simulink model "VehicleDynamicsModel"  (R2018a)
settings: Solver=ode15s  StartTime=0.0  StopTime=12  FixedStep=0.01  RelTol=1e-2  EnableMultiTasking=on
PreLoadFcn:
  | PowerTrain_14DOF_ini
StopFcn:
  | AfterSim
undefined symbols (not defined in the file): AccelCmd2TrqCmd, Chasis, GearRatio, Motor, Motor_J, Motor_RotorDamping, VEH, X, Y, Z
libraries: sm_lib x186, autolibutils x40, nesl_utility x23, vehdynlibtire x4, fuzblock x3, sharedtransform x2, autolibmappedmotorcommon x2, vehdynlibeom x1, vehdynlibsuspension x1, simulink x1, vehdynlibsteering x1
(part 2 of 11)

== system VehicleDynamicsModel/E23/14DOF/14DOF/Tires&Wheels/VDBS ==
  note: 魔术公式系数
      | （27行4列的矩阵）
  note: 魔术公式系数
  note: 转矩
      | 内倾角
      | 横摆角速度
      | 转向角
      | 速度到车轮坐标系的转化
  note: 横摆角速度
      |
      | 转矩
      |
      | 刹车压力
      |
      | 内倾角
      |
      | 车轮转向角
      |
      | 质心速度(车身
      | 坐标系）
  note: 轮胎对车身的反作
      | 用力
  note: 四个车轮，盘刹，
      | 考虑侧倾，横摆
  note: 悬架的作用力
  WheelAng : Inport
  CamberAng : Inport  Port=2
  AxleTrq : Inport  Port=3
  BrkPrs : Inport  Port=4
  Fz : Inport  Port=5
  r : Inport  Port=6
  VehVel : Inport  Port=7
  GroundLevel : Inport  Port=8
  Friction : Inport  Port=9
  4Wheels : Subsystem
  Pressure : Constant  Value=224006.174898101*ones(4,1)
  Terminator : Terminator
  Tires2Veh : Subsystem
  Veh2Tire : Subsystem
  scale factors with friction1 : Subsystem  mask{numWheels=4}
      mask prompts: numWheels "Number of wheels"
  Wheels : Outport
  FL : Outport  Port=2
  WhlOmega : Outport  Port=3
  FR : Outport  Port=4
  SuspWhlPz : Outport  Port=5
  SuspWhlVz : Outport  Port=6
  SteerTrq : Outport  Port=7
  wires:
  WheelAng/1 -> Tires2Veh/2(WheelSteer), Veh2Tire/5(Steer)
  BrkPrs/1 -> Veh2Tire/3(Braker)
  Tires2Veh/2(FL) -> FL/1
  Tires2Veh/1(Wheels) -> Wheels/1
  Veh2Tire/6(zdotAxle) -> Terminator/1
  Tires2Veh/5(SuspWhlPz) -> SuspWhlPz/1
  scale factors with friction1/1(lambdas) -> 4Wheels/8(lambda)
  r/1 -> Veh2Tire/1(r)
  CamberAng/1 -> Tires2Veh/3(WheelCamber), Veh2Tire/4(Camber), 4Wheels/6(Camber)
  Friction/1 -> scale factors with friction1/2(lamda_mu_y), scale factors with friction1/1(lamda_mu_x)
  Tires2Veh/3("WhlOmega ") -> WhlOmega/1
  Tires2Veh/4(FR) -> FR/1
  Pressure/1 -> 4Wheels/7(Press)
  Tires2Veh/6(SuspWhlVz) -> SuspWhlVz/1
  Fz/1 -> 4Wheels/10(FzSusp), Tires2Veh/4(Fz)
  Veh2Tire/3(psidot) -> 4Wheels/3(r)
  VehVel/1 -> Veh2Tire/6(VelVeh)
  AxleTrq/1 -> Veh2Tire/2(Axle)
  Veh2Tire/2(P) -> 4Wheels/2(BrakePressure)
  4Wheels/1(Wheels) -> Tires2Veh/1(Wheel)
  Veh2Tire/1(T) -> 4Wheels/1(DriveTorqe)
  Veh2Tire/5(ydotAxle) -> 4Wheels/5(Vy)
  Veh2Tire/4(xdotAxle) -> 4Wheels/4(Vx)
  GroundLevel/1 -> 4Wheels/9(Gnd)
  Tires2Veh/7(Mz) -> SteerTrq/1

== system VehicleDynamicsModel/E23/PowerTrain/DriveTrain/DriveLine/BrkPrs ==
  BrkPrsCmd : Inport
  Constant : Constant  Value=-1
  Gain1 : Gain  Gain=Chasis.MaxBrkPrs
  Switch : Switch  Criteria=u2 ~= 0
  Volume : Integrator  LimitOutput=on  UpperSaturationLimit=1  LowerSaturationLimit=0
  BrkPrs : Outport
  wires:
  Constant/1 -> Switch/3
  Gain1/1 -> BrkPrs/1
  Switch/1 -> Volume/1
  BrkPrsCmd/1 -> Switch/2, Switch/1
  Volume/1 -> Gain1/1

== system VehicleDynamicsModel/E23/PowerTrain/PowerTrain/MotorRL/Motor ==
  TrqCmd : Inport
  BattVolt : Inport  Port=2
  MtrSpd : Inport  Port=3
  Constant : Constant  Value=0
  Divide : Product  Inputs=*/
  Motor : Subsystem
      mask Display: image('Motor.jpg');
  Saturation : Saturate  UpperLimit=6e4  LowerLimit=1
  Scope : Scope  NumInputPorts=4
  Switch : Switch  Criteria=u2 > Threshold
  MechPwr : Outport
  Efficiency : Outport  Port=2
  MtrTrq : Outport  Port=3
  wires:
  TrqCmd/1 -> Motor/1(TrqCmd)
  BattVolt/1 -> Motor/2(BattVolt)
  Motor/1(MechPwr) -> [MechPwr], Scope/1  "MechPwr"
  Divide/1 -> Switch/1
  Motor/2(BattCurr) -> Scope/2  "BattCurr"
  [MechPwr] -> Switch/2, MechPwr/1, Divide/1
  Motor/3(MtrTrq) -> Scope/3, [MtrTrq]  "MtrTrq"
  [MtrTrq] -> MtrTrq/1
  [P_in] -> Saturation/1
  Saturation/1 -> Divide/2
  Switch/1 -> Efficiency/1
  Constant/1 -> Switch/3
  MtrSpd/1 -> Scope/4, Motor/3(MtrSpd)
  Motor/4(P_in) -> [P_in]

== system VehicleDynamicsModel/E23/PowerTrain/PowerTrain/MotorRR/Motor ==
  TrqCmd : Inport
  BattVolt : Inport  Port=2
  MtrSpd : Inport  Port=3
  Constant : Constant  Value=0
  Divide : Product  Inputs=*/
  Motor : Subsystem
      mask Display: image('Motor.jpg');
  Saturation : Saturate  UpperLimit=6e4  LowerLimit=1
  Scope : Scope  NumInputPorts=3
  Switch : Switch  Criteria=u2 > Threshold
  MechPwr : Outport
  Efficiency : Outport  Port=2
  MtrTrq : Outport  Port=3
  wires:
  TrqCmd/1 -> Motor/1(TrqCmd)
  BattVolt/1 -> Motor/2(BattVolt)
  Motor/1(MechPwr) -> [MechPwr], Scope/1  "MechPwr"
  Divide/1 -> Switch/1
  Motor/2(BattCurr) -> Scope/2  "BattCurr"
  [MechPwr] -> Switch/2, MechPwr/1, Divide/1
  Motor/3(MtrTrq) -> Scope/3, [MtrTrq]  "MtrTrq"
  [MtrTrq] -> MtrTrq/1
  [P_in] -> Saturation/1
  Saturation/1 -> Divide/2
  Switch/1 -> Efficiency/1
  Constant/1 -> Switch/3
  MtrSpd/1 -> Motor/3(MtrSpd)
  Motor/4(P_in) -> [P_in]

== system VehicleDynamicsModel/E23/14DOF/14DOF/Suspension/ChasisWhlAngs/Variant Subsystem ==
  note: 1) Add Subsystem or Model blocks as valid variant choices.
      | 2) You cannot connect blocks at this level. At simulation, connectivity is automatically
      | determined, based on the active variant and port name matching.
  FxR : Inport
  FyR : Inport  Port=2
  FzR : Inport  Port=3
  Debug : Subsystem  VariantControl=Variant
  Release : Subsystem  VariantControl=Variant1
  WhlAng : Outport

== system VehicleDynamicsModel/E23/14DOF/14DOF/Suspension/UseMultibody/No ==
  Camber : Inport
  CasterToe : Inport  Port=2
  Steering : Inport  Port=3
  Constant : Constant  Value=zeros(3,4)
  Matrix Sum : Sum
  Terminator : Terminator
  Terminator1 : Terminator
  Terminator2 : Terminator
  WhlAng : Outport
  wires:
  Camber/1 -> Terminator/1
  CasterToe/1 -> Terminator1/1
  Steering/1 -> Matrix Sum/2, Terminator2/1
  Constant/1 -> Matrix Sum/1
  Matrix Sum/1 -> WhlAng/1

== system VehicleDynamicsModel/E23/14DOF/14DOF/Suspension/UseMultibody/Yes ==
  Camber : Inport
  CasterToe : Inport  Port=2
  Steering : Inport  Port=3
  Matrix Sum : Sum  Inputs=+++
  WhlAng : Outport
  wires:
  Camber/1 -> Matrix Sum/1
  CasterToe/1 -> Matrix Sum/2
  Matrix Sum/1 -> WhlAng/1
  Steering/1 -> Matrix Sum/3
